simulink model "HW4_2"  (R2023a)
settings: Solver=VariableStepAuto  StartTime=0.0  StopTime=10.0  RelTol=1e-3
settings Model: Creator=BRL  LastModifiedBy=BRL

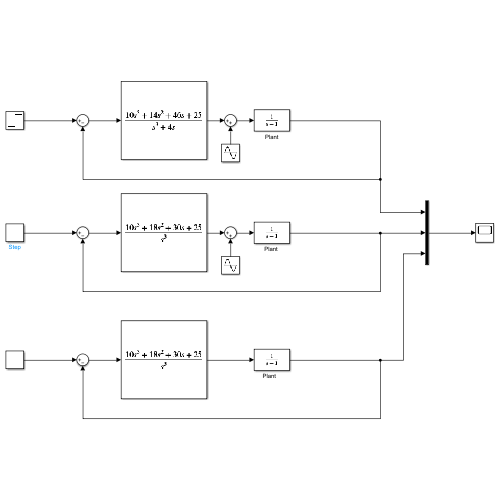
[thumbnail: Simulink's stored preview of the top-level diagram]
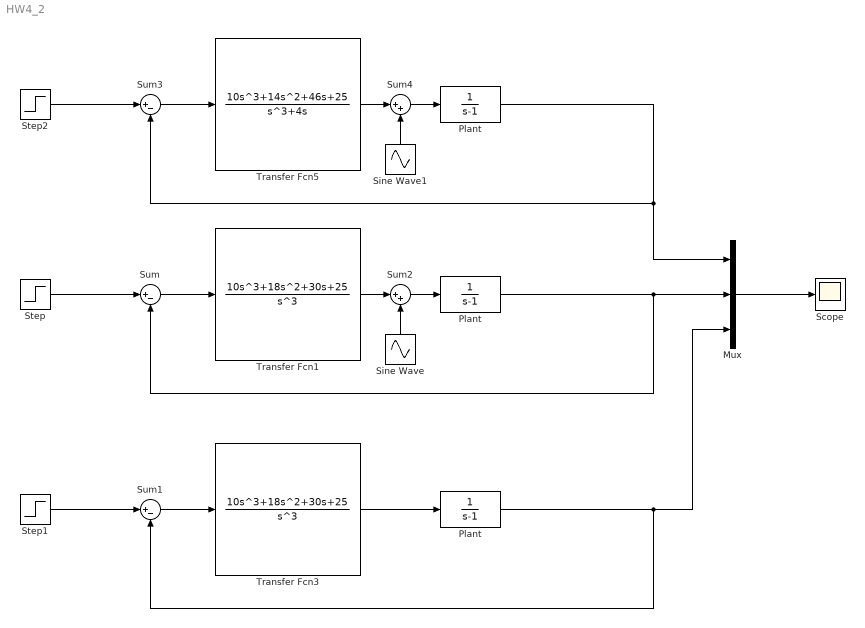
== system HW4_2 ==
  Mux : Mux  Inputs=3
  Plant : TransferFcn  Denominator=[1 -1]
  "Plant " : TransferFcn  Denominator=[1 -1]
  "Plant   " : TransferFcn  Denominator=[1 -1]
  Scope : Scope
  Sine Wave : Sin  Frequency=2  Phase=pi/6  SampleTime=0
  Sine Wave1 : Sin  Frequency=2  Phase=pi/6  SampleTime=0
  Step : Step  SampleTime=0
  Step1 : Step  SampleTime=0
  Step2 : Step  SampleTime=0
  Sum : Sum  Inputs=|+-
  Sum1 : Sum  Inputs=|+-
  Sum2 : Sum  Inputs=|++
  Sum3 : Sum  Inputs=|+-
  Sum4 : Sum  Inputs=|++
  Transfer Fcn1 : TransferFcn  Numerator=[10 18 30 25]  Denominator="[1 0  0 0]"
  Transfer Fcn3 : TransferFcn  Numerator=[10 18 30 25]  Denominator="[1 0  0 0]"
  Transfer Fcn5 : TransferFcn  Numerator=[10 14 46 25]  Denominator="[1 0  4 0]"
  wires:
  Step/1 -> Sum/1
  Sum/1 -> Transfer Fcn1/1
  Transfer Fcn3/1 -> "Plant   "/1
  Step1/1 -> Sum1/1
  "Plant   "/1 -> Mux/3, Sum1/2
  Sum1/1 -> Transfer Fcn3/1
  "Plant "/1 -> Mux/2, Sum/2
  Sum2/1 -> "Plant "/1
  Sine Wave/1 -> Sum2/2
  Transfer Fcn1/1 -> Sum2/1
  Mux/1 -> Scope/1
  Transfer Fcn5/1 -> Sum4/1
  Sum3/1 -> Transfer Fcn5/1
  Sine Wave1/1 -> Sum4/2
  Step2/1 -> Sum3/1
  Plant/1 -> Mux/1, Sum3/2
  Sum4/1 -> Plant/1
